simulink model "CT_xbee_2010a"  (Simulink 8.1)
settings: Solver=ode45  StartTime=0.0  StopTime=60  FixedStep=Tm  RelTol=1e-3
InitFcn:
  | Tm = 0.1;
undefined symbols (not defined in the file or in its folder): A, B
libraries: simulink x6
settings Model: Creator=Equipo-Servo  LastModifiedBy=Equipo-Servo  ExtModeTrigDuration=100000
settings OptimizationCC: ExpressionDepthLimit=128
settings DebuggingCC: FcnCallInpInsideContextMsg=EnableAllAsWarning
settings HardwareCC: ProdIntDivRoundTo=Zero  ProdEndianess=LittleEndian  ProdHWDeviceType=Generic->32-bit x86 compatible
settings RTWCC: SystemTargetFile=rtwin.tlc  TemplateMakefile=rtwin.tmf  Description=Real-Time Windows Target  ProcessScript=rtwin_make_rtw_hook  RTWCompilerOptimization=On
settings CodeAppCC: MaxIdLength=95
settings RTWinTargetCC: TargetLibSuffix=_rtwin.lib  TargetPreCompLibLocation=C:\Program Files\MATLAB\R2013a\toolbox\rtw\targets\rtwin\lib\win32  CodeReplacementLibrary=ANSI_C  MatFileLogging=on  RTWinDir=C:/PROGRA~1/MATLAB/R2013a/toolbox/rtw/targets/rtwin  TargetArch=win32

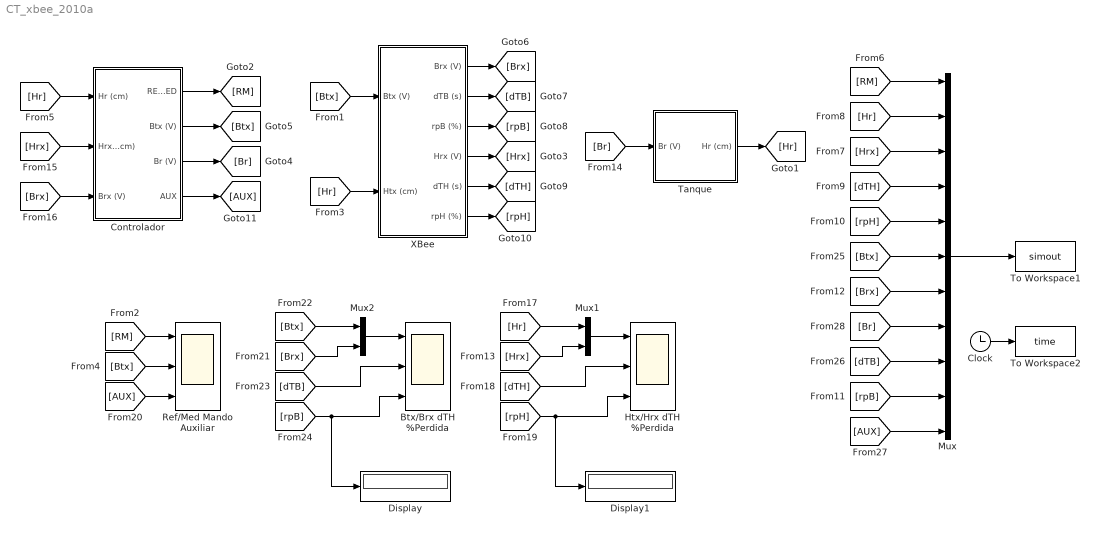
== system CT_xbee_2010a ==
  Btx/Brx dTH %Perdida : Scope  NumInputPorts=3
      settings: TimeRange=60  YMin=0~0~0  YMax=5~0.4~80  SaveName=ScopeData2
  Clock : Clock
  Controlador : Subsystem
  Display : Display
  Display1 : Display
  Htx/Hrx dTH %Perdida : Scope  NumInputPorts=3
      settings: TimeRange=60  YMin=-5~0~0  YMax=20~0.5~80
  Mux : Mux  Inputs=11
  Mux1 : Mux  Inputs=2
  Mux2 : Mux  Inputs=2
  Ref/Med Mando Auxiliar : Scope  NumInputPorts=3
      settings: TimeRange=60  YMin=-5~0~-5  YMax=20~5~20
  Tanque : Subsystem
  To Workspace1 : ToWorkspace  VariableName=simout  SampleTime=Tm  SaveFormat=Structure With Time
  To Workspace2 : ToWorkspace  VariableName=time  SampleTime=Tm
  XBee : Subsystem
  wires:
  Mux/1 -> To Workspace1/1
  Clock/1 -> To Workspace2/1
  [RM] -> Mux/1
  [Hr] -> Mux/2
  [Hrx] -> Mux/3
  [dTH] -> Mux/4
  [rpH] -> Mux/5
  Controlador/1(REF/MED) -> [RM]
  Controlador/2(Btx (V)) -> [Btx]
  [Br] -> Tanque/1(Br (V))
  Tanque/1(Hr (cm)) -> [Hr]
  [Btx] -> XBee/1(Btx (V))
  [Hr] -> XBee/2(Htx (cm))
  [Hr] -> Controlador/1(Hr (cm))
  XBee/4(Hrx (V)) -> [Hrx]
  [Hrx] -> Controlador/2(Hrx (cm))
  XBee/1(Brx (V)) -> [Brx]
  XBee/2(dTB (s)) -> [dTB]
  XBee/3(rpB (%)) -> [rpB]
  XBee/5(dTH (s)) -> [dTH]
  XBee/6(rpH (%)) -> [rpH]
  [Brx] -> Controlador/3(Brx (V))
  [RM] -> Ref/Med Mando Auxiliar/1
  [Btx] -> Ref/Med Mando Auxiliar/2
  [Hr] -> Mux1/1
  [Hrx] -> Mux1/2
  Mux1/1 -> Htx/Hrx dTH %Perdida/1
  [AUX] -> Ref/Med Mando Auxiliar/3
  [Btx] -> Mux2/1
  [Brx] -> Mux2/2
  Mux2/1 -> Btx/Brx dTH %Perdida/1
  Controlador/3(Br (V)) -> [Br]
  Controlador/4(AUX) -> [AUX]
  [Btx] -> Mux/6
  [Brx] -> Mux/7
  [dTH] -> Htx/Hrx dTH %Perdida/2
  [rpH] -> Display1/1, Htx/Hrx dTH %Perdida/3
  [dTB] -> Btx/Brx dTH %Perdida/2
  [rpB] -> Display/1, Btx/Brx dTH %Perdida/3
  [AUX] -> Mux/11
  [rpB] -> Mux/10
  [dTB] -> Mux/9
  [Br] -> Mux/8

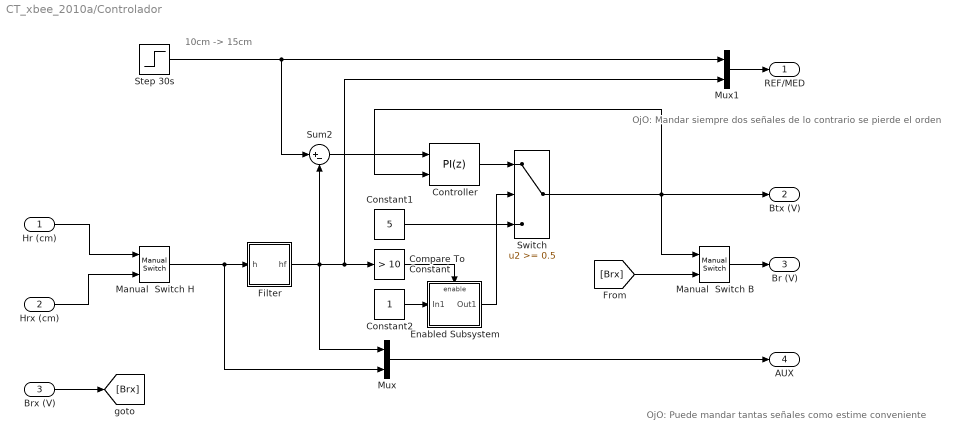
== system CT_xbee_2010a/Controlador ==
  note: 10cm -> 15cm
  note: OjO: Mandar siempre dos señales
      | de lo contrario se pierde el orden
  note: OjO: Puede mandar tantas señales
      | como estime conveniente
  Hr (cm) : Inport
  Hrx (cm) : Inport  Port=2
  Brx (V) : Inport  Port=3
  Compare To Constant : simulink/Logic and Bit Operations/Compare To Constant  relop=>  const=10  LogicOutDataTypeMode=boolean
  Constant1 : Constant  Value=5
  Constant2 : Constant
  Controller : simulink/Continuous/PID Controller  Controller=PI  TimeDomain=Discrete-time  SampleTime=Tm  IntegratorMethod=Forward Euler  FilterMethod=Forward Euler  Form=Parallel  P=3  I=1  D=0  N=100  InitialConditionSource=internal  InitialConditionForIntegrator=0  InitialConditionForFilter=0  ExternalReset=none  LimitOutput=on  UpperSaturationLimit=5  LowerSaturationLimit=0  LinearizeAsGain=off  AntiWindupMode=back-calculation  Kb=1  TrackingMode=on  Kt=1  PParamMin=[]  PParamMax=[]  IParamMin=[]  IParamMax=[]  DParamMin=[]  DParamMax=[]  NParamMin=[]  NParamMax=[]  KbParamMin=[]  KbParamMax=[]  KtParamMin=[]  KtParamMax=[]  POutMin=[]  POutMax=[]  IOutMin=[]  IOutMax=[]  DOutMin=[]  DOutMax=[]  NOutMin=[]  NOutMax=[]  KbOutMin=[]  KbOutMax=[]  KtOutMin=[]  KtOutMax=[]  IntegratorOutMin=[]  IntegratorOutMax=[]  FilterOutMin=[]  FilterOutMax=[]  SumOutMin=[]  SumOutMax=[]  SumI1OutMin=[]  SumI1OutMax=[]  SumI2OutMin=[]  SumI2OutMax=[]  SumI3OutMin=[]  SumI3OutMax=[]  SumDOutMin=[]  SumDOutMax=[]  SaturationOutMin=[]  SaturationOutMax=[]  IntegratorContinuousStateAttributes=''  IntegratorStateMustResolveToSignalObject=off  IntegratorRTWStateStorageClass=Auto  FilterContinuousStateAttributes=''  FilterStateMustResolveToSignalObject=off  FilterRTWStateStorageClass=Auto
  Enabled Subsystem : Subsystem  TreatAsAtomicUnit=on
  Filter : Subsystem  mask{O=2, Fc=0.5, Tm=Tm}
      mask prompts: O "Orden"; Fc "Frecuencia de corte"; Tm "Periodo de muestreo"
      mask init:
      | Fm = 1/Tm;
      | [B,A] = butter(O,Fc/(Fm/2));
  Manual  Switch B : simulink/Signal Routing/Manual Switch  sw=0  action=0  varsize=off
  Manual  Switch H : simulink/Signal Routing/Manual Switch  sw=0  action=0  varsize=off
  Mux : Mux  Inputs=2
  Mux1 : Mux  Inputs=2
  Step 30s : Step  Time=30  Before=10  After=15  SampleTime=0
  Sum2 : Sum  Inputs=|+-
  Switch : Switch  Threshold=0.5
  REF/MED : Outport
  Btx (V) : Outport  Port=2
  Br (V) : Outport  Port=3
  AUX : Outport  Port=4
  wires:
  Enabled Subsystem/1(Out1) -> Switch/2
  Sum2/1 -> Controller/1
  Constant2/1 -> Enabled Subsystem/1(In1)
  Compare To Constant/1 -> Enabled Subsystem/Enable
  Constant1/1 -> Switch/3
  Controller/1 -> Switch/1
  Filter/1(hf) -> Mux/1, Sum2/2, Mux1/2, Compare To Constant/1
  Step 30s/1 -> Sum2/1, Mux1/1
  Manual  Switch H/1 -> Filter/1(h), Mux/2
  Hr (cm)/1 -> Manual  Switch H/1
  Hrx (cm)/1 -> Manual  Switch H/2
  Brx (V)/1 -> [Brx]
  [Brx] -> Manual  Switch B/2
  Mux1/1 -> REF/MED/1
  Switch/1 -> Manual  Switch B/1, Controller/2, Btx (V)/1
  Mux/1 -> AUX/1
  Manual  Switch B/1 -> Br (V)/1

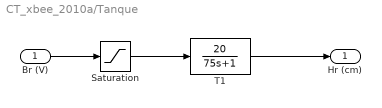
== system CT_xbee_2010a/Tanque ==
  Br (V) : Inport
  Saturation : Saturate  UpperLimit=5  LowerLimit=0
  T1 : TransferFcn  Numerator=[20]  Denominator=[75 1]
  Hr (cm) : Outport
  wires:
  T1/1 -> Hr (cm)/1
  Br (V)/1 -> Saturation/1
  Saturation/1 -> T1/1

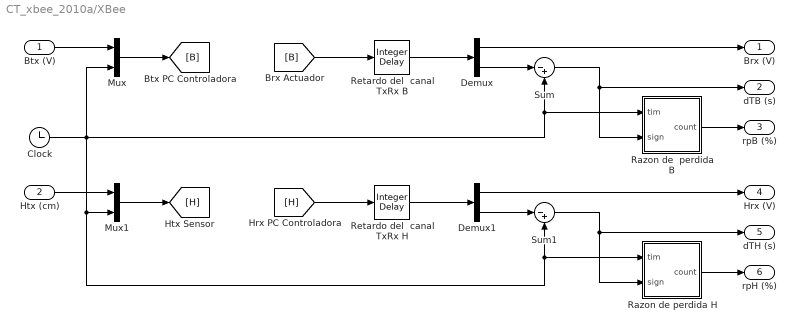
== system CT_xbee_2010a/XBee ==
  Btx (V) : Inport
  Htx (cm) : Inport  Port=2
  Clock : Clock
  Demux : Demux  Outputs=2
  Demux1 : Demux  Outputs=2
  Mux : Mux  Inputs=2
  Mux1 : Mux  Inputs=2
  Razon de perdida H : Subsystem  mask{Ttx=Tm}
  Razon de  perdida B : Subsystem  mask{Ttx=Tm}
  Retardo del  canal TxRx B : simulink/Discrete/Integer Delay  NumDelays=1  vinit=0.0  samptime=Tm
  Retardo del  canal TxRx H : simulink/Discrete/Integer Delay  NumDelays=1  vinit=0.0  samptime=Tm
  Sum : Sum  Inputs=|-+
  Sum1 : Sum  Inputs=|-+
  Brx (V) : Outport
  dTB (s) : Outport  Port=2
  rpB (%) : Outport  Port=3
  Hrx (V) : Outport  Port=4
  dTH (s) : Outport  Port=5
  rpH (%) : Outport  Port=6
  wires:
  Btx (V)/1 -> Mux/1
  Mux/1 -> [B]
  Demux/2 -> Sum/1
  Sum/1 -> dTB (s)/1, Razon de  perdida B/2(sign)
  Demux/1 -> Brx (V)/1
  Razon de  perdida B/1(count) -> rpB (%)/1
  Htx (cm)/1 -> Mux1/1
  Clock/1 -> Mux/2, Sum/2, Razon de  perdida B/1(tim), Razon de perdida H/1(tim), Sum1/2, Mux1/2
  Mux1/1 -> [H]
  [H] -> Retardo del  canal TxRx H/1
  Demux1/2 -> Sum1/1
  Sum1/1 -> Razon de perdida H/2(sign), dTH (s)/1
  Demux1/1 -> Hrx (V)/1
  Razon de perdida H/1(count) -> rpH (%)/1
  Retardo del  canal TxRx B/1 -> Demux/1
  [B] -> Retardo del  canal TxRx B/1
  Retardo del  canal TxRx H/1 -> Demux1/1

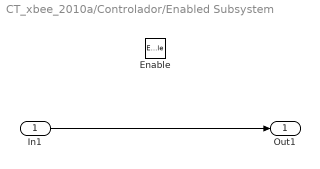
== system CT_xbee_2010a/Controlador/Enabled Subsystem ==
  In1 : Inport
  Enable : EnablePort
  Out1 : Outport
  wires:
  In1/1 -> Out1/1

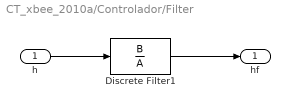
== system CT_xbee_2010a/Controlador/Filter ==
  h : Inport
  Discrete Filter1 : DiscreteFilter  Numerator=B  Denominator=A  SampleTime=Tm
  hf : Outport
  wires:
  h/1 -> Discrete Filter1/1
  Discrete Filter1/1 -> hf/1

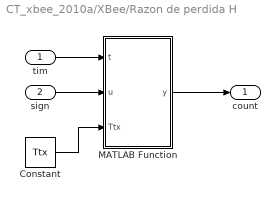
== system CT_xbee_2010a/XBee/Razon de perdida H ==
  tim : Inport
  sign : Inport  Port=2
  Constant : Constant  Value=Ttx
  MATLAB Function : MATLAB Function  TreatAsAtomicUnit=on
  count : Outport
  wires:
  Constant/1 -> MATLAB Function/3(Ttx)
  MATLAB Function/1(y) -> count/1
  tim/1 -> MATLAB Function/1(t)
  sign/1 -> MATLAB Function/2(u)

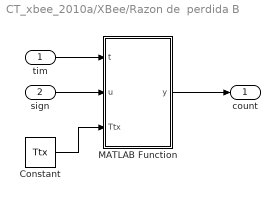
== system CT_xbee_2010a/XBee/Razon de  perdida B ==
  tim : Inport
  sign : Inport  Port=2
  Constant : Constant  Value=Ttx
  MATLAB Function : MATLAB Function  TreatAsAtomicUnit=on
  count : Outport
  wires:
  sign/1 -> MATLAB Function/2(u)
  tim/1 -> MATLAB Function/1(t)
  MATLAB Function/1(y) -> count/1
  Constant/1 -> MATLAB Function/3(Ttx)

== matlab function XBee/Razon de perdida H/MATLAB Function ==
  data: t input double; u input double; y output double; Ttx input double
function y = fcn(t,u,Ttx)

u = round(u*100)/100;

persistent u1 c i

if isempty(u1)
    u1 = u;
    c = 0;
    i = 1;
end

if (t>i*Ttx)
    i = i + 1;
    %if ((u > u1) || ((u>Ttx)&&(u==u1)))
    if (u > u1)
        c = c + 1;
    end
    u1 = u;
end

y = 100*c/i;

== matlab function XBee/Razon de perdida B/MATLAB Function ==
  data: t input double; u input double; y output double; Ttx input double
function y = fcn(t,u,Ttx)

u = round(u*100)/100;

persistent u1 c i

if isempty(u1)
    u1 = u;
    c = 0;
    i = 1;
end

if (t>i*Ttx)
    i = i + 1;
    %if ((u > u1) || ((u>Ttx)&&(u==u1)))
    if (u > u1)
        c = c + 1;
    end
    u1 = u;
end

y = 100*c/i;
